simulink model "practica2"  (R2017b)
settings: Solver=VariableStepAuto  StartTime=0.0  StopTime=10  RelTol=1e-3
settings Model: Creator=DELL-PC  LastModifiedBy=DELL-PC

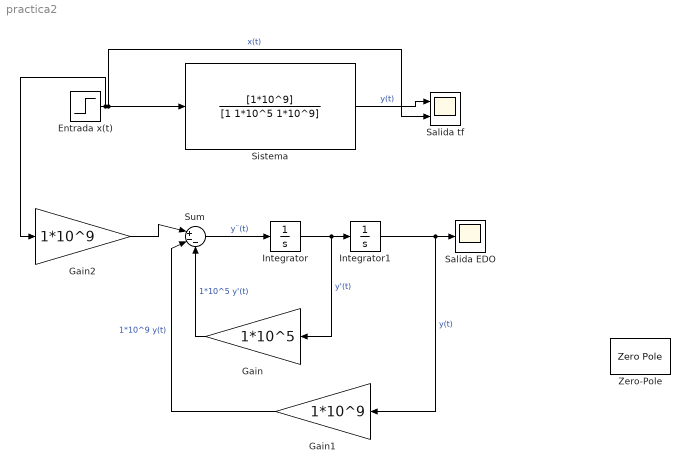
== system practica2 ==
  Entrada x(t) : Step  Time=0  After=5  SampleTime=0
  "Gain " : Gain  Gain=1*10^5
  "Gain1 " : Gain  Gain=1*10^9
  "Gain2 " : Gain  Gain=1*10^9
  "Integrator " : Integrator
  "Integrator1 " : Integrator
  Salida EDO : Scope
  Salida tf : Scope  NumInputPorts=2
  Sistema : TransferFcn  Numerator=[1*10^9]  Denominator=[1 1*10^5 1*10^9]
  Sum : Sum  Inputs=|+--
  Zero-Pole : ZeroPole  Poles=[0 -1]
  wires:
  Sistema/1 -> Salida tf/1  "y(t)"
  Sum/1 -> "Integrator "/1  "y¨(t)"
  "Integrator1 "/1 -> Salida EDO/1, "Gain1 "/1  "y(t)"
  "Gain "/1 -> Sum/3  "1*10^5 y'(t)"
  "Integrator "/1 -> "Gain "/1, "Integrator1 "/1  "y'(t)"
  "Gain1 "/1 -> Sum/2  "1*10^9 y(t)"
  "Gain2 "/1 -> Sum/1
  Entrada x(t)/1 -> "Gain2 "/1, Salida tf/2, Sistema/1  "x(t)"
